simulink model "AStar_Obstacle_Fix_Offset"  (R2019a)
settings: Solver=FixedStepAuto  StartTime=0.0  StopTime=inf  FixedStep=0.1  RelTol=1e-3
undefined symbols (not defined in the file): Angular, Linear
libraries: robotlib x4, simulink x1
settings Model: Creator=user  LastModifiedBy=user
settings OptimizationCC: EnhancedBackFolding=on  PassReuseOutputArgsAs=Individual arguments  MaxStackSize=64  OptimizeBlockOrder=speed  DifferentSizesBufferReuse=on  OptimizationCustomize=off
settings DebuggingCC: ParameterTunabilityLossMsg=error
settings HardwareCC: ProdBitPerPointer=32  ProdBitPerSizeT=32  ProdBitPerPtrDiffT=32  ProdLargestAtomicFloat=None  ProdIntDivRoundTo=Undefined  ProdEndianess=Unspecified  ProdWordSize=32  ProdHWDeviceType=Generic->Unspecified (assume 32-bit Generic)
settings SFSimCC: MATLABDynamicMemAlloc=off
settings RTWCC: SystemTargetFile=ert.tlc  HardwareBoard=Robot Operating System (ROS)  TLCOptions="-aInlineSetEventsForThisBaseRateFcn=TLC_FALSE -aSuppressMultiTaskScheduler=TLC_FALSE  -aRateBasedStepFcn=0"  TemplateMakefile=ert_default_tmf  GenerateReport=on  Toolchain=Catkin  IncludeHyperlinkInReport=on  LaunchReport=on  TargetLang=C++  GenerateTraceInfo=on  GenerateTraceReport=on  GenerateTraceReportSl=on  GenerateTraceReportSf=on  GenerateTraceReportEml=on
settings CodeAppCC: ForceParamTrailComments=on  IgnoreCustomStorageClasses=off  OperatorAnnotations=on  SimulinkDataObjDesc=on  SFDataObjDesc=on  InsertBlockDesc=on

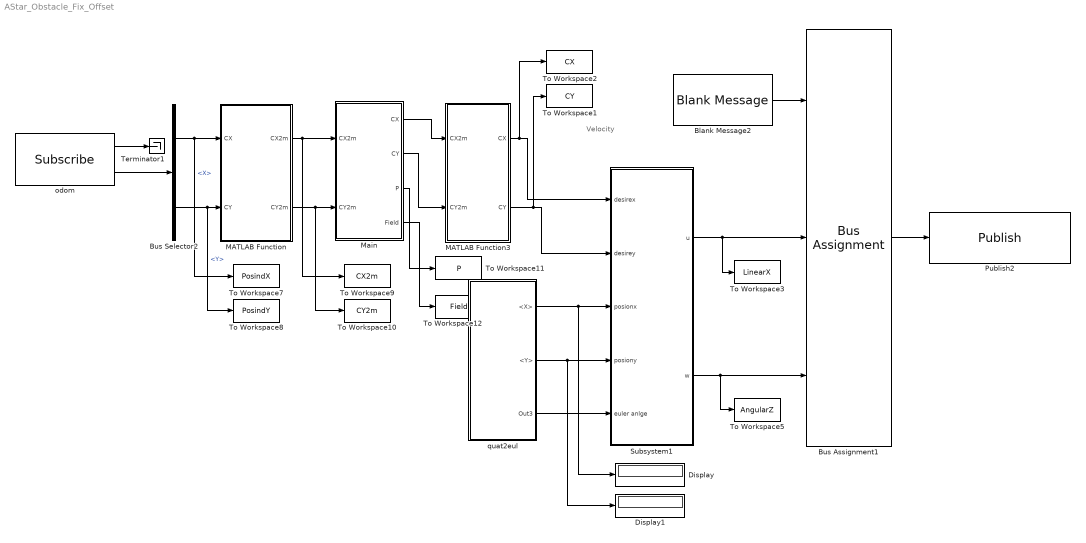
== system AStar_Obstacle_Fix_Offset ==
  note: Velocity
  Blank Message2 : robotlib/Blank Message  messageClass=Message  entityType=geometry_msgs/Twist  messageType=geometry_msgs/Twist  SampleTime=inf
      settings: SourceProductBaseCode=RO
  Bus Assignment1 : BusAssignment  AssignedSignals=Linear.X,Angular.Z
  Bus Selector2 : BusSelector  OutputSignals=Pose.Pose.Position.X,Pose.Pose.Position.Y
  Display : Display
  Display1 : Display
  MATLAB Function : MATLAB Function  TreatAsAtomicUnit=on
  MATLAB Function3 : MATLAB Function  TreatAsAtomicUnit=on
  Main : MATLAB Function  TreatAsAtomicUnit=on
  Publish2 : robotlib/Publish  topicSource=Select from ROS network  topic=/cmd_vel  messageType=geometry_msgs/Twist  messageQueueLength=1
      settings: SourceProductBaseCode=RO
  Subsystem1 : Subsystem
  Terminator1 : Terminator
  To Workspace1 : ToWorkspace  VariableName=CY  SampleTime=-1
      settings: Save2DSignal=2-D array (concatenate along first dimension)
  To Workspace10 : ToWorkspace  VariableName=CY2m  SampleTime=-1
      settings: Save2DSignal=2-D array (concatenate along first dimension)
  To Workspace11 : ToWorkspace  VariableName=P  SampleTime=-1
      settings: Save2DSignal=2-D array (concatenate along first dimension)
  To Workspace12 : ToWorkspace  VariableName=Field  SampleTime=-1
      settings: Save2DSignal=2-D array (concatenate along first dimension)
  To Workspace2 : ToWorkspace  VariableName=CX  SampleTime=-1
      settings: Save2DSignal=2-D array (concatenate along first dimension)
  To Workspace3 : ToWorkspace  VariableName=LinearX  SampleTime=-1
      settings: Save2DSignal=2-D array (concatenate along first dimension)
  To Workspace5 : ToWorkspace  VariableName=AngularZ  SampleTime=-1
      settings: Save2DSignal=2-D array (concatenate along first dimension)
  To Workspace7 : ToWorkspace  VariableName=PosindX  SampleTime=-1
      settings: Save2DSignal=2-D array (concatenate along first dimension)
  To Workspace8 : ToWorkspace  VariableName=PosindY  SampleTime=-1
      settings: Save2DSignal=2-D array (concatenate along first dimension)
  To Workspace9 : ToWorkspace  VariableName=CX2m  SampleTime=-1
      settings: Save2DSignal=2-D array (concatenate along first dimension)
  odom : robotlib/Subscribe  topicSource=Select from ROS network  topic=/odom  messageType=nav_msgs/Odometry  sampleTime=-1  messageQueueLength=1
      settings: SourceProductBaseCode=RO
  quat2eul : Subsystem
  wires:
  MATLAB Function/1(CX2m) -> To Workspace9/1, Main/1(CX2m)
  MATLAB Function/2(CY2m) -> To Workspace10/1, Main/2(CY2m)
  odom/1 -> Terminator1/1
  Main/1(CX) -> MATLAB Function3/1(CX2m)
  Main/2(CY) -> MATLAB Function3/2(CY2m)
  odom/2 -> Bus Selector2/1
  Bus Selector2/1 -> To Workspace7/1, MATLAB Function/1(CX)  "<X>"
  Bus Selector2/2 -> To Workspace8/1, MATLAB Function/2(CY)  "<Y>"
  Subsystem1/2(w) -> To Workspace5/1, Bus Assignment1/3
  quat2eul/2(<Y>) -> Display1/1, Subsystem1/4(posiony)
  MATLAB Function3/1(CX) -> To Workspace2/1, Subsystem1/1(desirex)
  MATLAB Function3/2(CY) -> To Workspace1/1, Subsystem1/2(desirey)
  quat2eul/1(<X>) -> Display/1, Subsystem1/3(posionx)
  Subsystem1/1(u) -> To Workspace3/1, Bus Assignment1/2
  quat2eul/3(Out3) -> Subsystem1/5(euler anlge)
  Bus Assignment1/1 -> Publish2/1
  Blank Message2/1 -> Bus Assignment1/1
  Main/3(P) -> To Workspace11/1
  Main/4(Field) -> To Workspace12/1

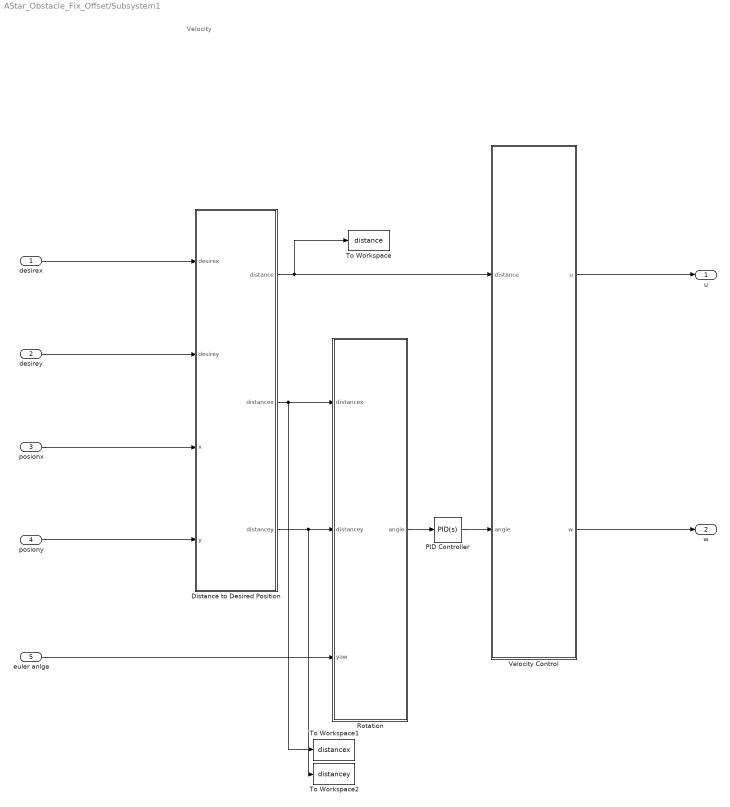
== system AStar_Obstacle_Fix_Offset/Subsystem1 ==
  note: Velocity
  desirex : Inport
  desirey : Inport  Port=2
  posionx : Inport  Port=3
  posiony : Inport  Port=4
  euler anlge : Inport  Port=5
  Distance to Desired Position : MATLAB Function  TreatAsAtomicUnit=on
  PID Controller : simulink/Continuous/PID Controller  Controller=PID  Form=Parallel  TimeDomain=Continuous-time  SampleTime=-1  IntegratorMethod=Forward Euler  FilterMethod=Forward Euler  ControllerParametersSource=internal  P=1.1  I=0  D=0  UseFilter=on  N=100  TunerSelectOption=Transfer Function Based (PID Tuner App)  InitialConditionSource=internal  InitialConditionForIntegrator=0  InitialConditionForFilter=0  DifferentiatorICPrevScaledInput=0  ExternalReset=none  TrackingMode=off  Kt=1  LimitOutput=off  UpperSaturationLimit=inf  LowerSaturationLimit=-inf  LinearizeAsGain=on  AntiWindupMode=none  Kb=1  POutMin=[]  POutMax=[]  IOutMin=[]  IOutMax=[]  DOutMin=[]  DOutMax=[]  NOutMin=[]  NOutMax=[]  SumOutMin=[]  SumOutMax=[]  SaturationOutMin=[]  SaturationOutMax=[]  PParamMin=[]  PParamMax=[]  IParamMin=[]  IParamMax=[]  DParamMin=[]  DParamMax=[]  NParamMin=[]  NParamMax=[]  KbParamMin=[]  KbParamMax=[]  KtParamMin=[]  KtParamMax=[]  KbOutMin=[]  KbOutMax=[]  KtOutMin=[]  KtOutMax=[]  IntegratorOutMin=[]  IntegratorOutMax=[]  FilterOutMin=[]  FilterOutMax=[]  SumI1OutMin=[]  SumI1OutMax=[]  SumI2OutMin=[]  SumI2OutMax=[]  SumI3OutMin=[]  SumI3OutMax=[]  SumI4OutMin=[]  SumI4OutMax=[]  SumDOutMin=[]  SumDOutMax=[]  DifferentiatorOutMin=[]  DifferentiatorOutMax=[]  FilterDiffOutCoefMin=[]  FilterDiffOutCoefMax=[]  ReciprocalOutMin=[]  ReciprocalOutMax=[]  SumDenOutMin=[]  SumDenOutMax=[]  SumNumOutMin=[]  SumNumOutMax=[]  DivideOutMin=[]  DivideOutMax=[]  IntegratorContinuousStateAttributes=''  IntegratorStateMustResolveToSignalObject=off  IntegratorRTWStateStorageClass=Auto  FilterContinuousStateAttributes=''  FilterStateMustResolveToSignalObject=off  FilterRTWStateStorageClass=Auto  ParallelPVariant=InternalParameters  IdealPVariant=Disabled  IVariant=InternalParameters  DVariant=InternalParameters  IntegratorVariant=Continuous  SatVariant=Disabled  AWVariant=Passthrough  PCopyVariant=Disabled  TRVariant=Disabled  FdbkBlocksVariant=Forward  IdealPFdbkVariant=Disabled  SatFdbkVariant=Disabled  DerivativeFilterVariant=ContFilter  NVariant=InternalParameters  NCopyVariant=Disabled  FilterICVariant=InternalICsFilter  IntegratorICVariant=InternalICs  ExternalResetVariant=Disabled  TRSumVariant=Passthrough  SumFdbkVariant=Disabled  SumVariant=Sum_PID
  Rotation : MATLAB Function  TreatAsAtomicUnit=on
  To Workspace : ToWorkspace  VariableName=distance  SampleTime=-1
      settings: Save2DSignal=2-D array (concatenate along first dimension)
  To Workspace1 : ToWorkspace  VariableName=distancex  SampleTime=-1
      settings: Save2DSignal=2-D array (concatenate along first dimension)
  To Workspace2 : ToWorkspace  VariableName=distancey  SampleTime=-1
      settings: Save2DSignal=2-D array (concatenate along first dimension)
  Velocity Control : MATLAB Function  TreatAsAtomicUnit=on
  u : Outport
  w : Outport  Port=2
  wires:
  desirex/1 -> Distance to Desired Position/1(desirex)
  desirey/1 -> Distance to Desired Position/2(desirey)
  Distance to Desired Position/2(distancex) -> To Workspace1/1, Rotation/1(distancex)
  Velocity Control/2(w) -> w/1
  posionx/1 -> Distance to Desired Position/3(x)
  euler anlge/1 -> Rotation/3(yaw)
  posiony/1 -> Distance to Desired Position/4(y)
  Rotation/1(angle) -> PID Controller/1
  PID Controller/1 -> Velocity Control/2(angle)
  Distance to Desired Position/1(distance) -> To Workspace/1, Velocity Control/1(distance)
  Velocity Control/1(u) -> u/1
  Distance to Desired Position/3(distancey) -> To Workspace2/1, Rotation/2(distancey)

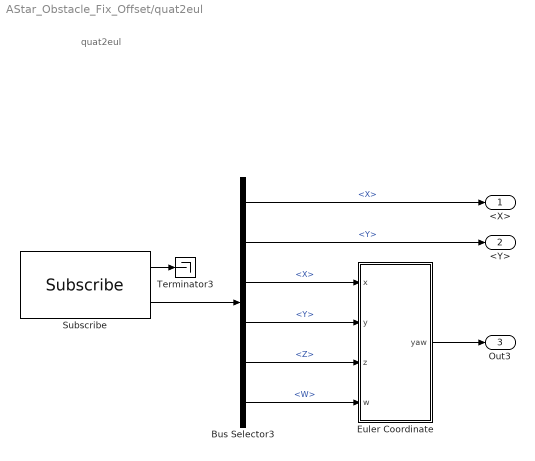
== system AStar_Obstacle_Fix_Offset/quat2eul ==
  note: quat2eul
  Bus Selector3 : BusSelector  OutputSignals=Pose.Pose.Position.X,Pose.Pose.Position.Y,Pose.Pose.Orientation.X,Pose.Pose.Orientation.Y,Pose.Pose.Orientation.Z,Pose.Pose.Orientation.W
  Euler Coordinate : MATLAB Function  TreatAsAtomicUnit=on
  Subscribe : robotlib/Subscribe  topicSource=Select from ROS network  topic=/odom  messageType=nav_msgs/Odometry  sampleTime=-1  messageQueueLength=1
      settings: SourceProductBaseCode=RO
  Terminator3 : Terminator
  <X> : Outport
  <Y> : Outport  Port=2
  Out3 : Outport  Port=3
  wires:
  Euler Coordinate/1(yaw) -> Out3/1
  Bus Selector3/5 -> Euler Coordinate/3(z)  "<Z>"
  Bus Selector3/6 -> Euler Coordinate/4(w)  "<W>"
  Subscribe/1 -> Terminator3/1
  Bus Selector3/3 -> Euler Coordinate/1(x)  "<X>"
  Subscribe/2 -> Bus Selector3/1
  Bus Selector3/4 -> Euler Coordinate/2(y)  "<Y>"
  Bus Selector3/2 -> <Y>/1  "<Y>"
  Bus Selector3/1 -> <X>/1  "<X>"

== matlab function AStar_Obstacle_Fix_Offset/quat2eul/Euler Coordinate ==
  data: x input; yaw output; y input; z input; w input
function yaw = quat2eul(x,y,z,w)

eul = quat2eul([w,x,y,z]);
yaw = eul(1);

end

== matlab function AStar_Obstacle_Fix_Offset/Main ==
  data: CX2m input; CY2m input; CX output; CY output; P output; Field output
function [CX,CY,P,Field] = astar(CX2m,CY2m)

N = 35;
Look = 0.04;
Offset = 50;

Start = [CY2m,CX2m]; % 반대로 줘야 함
Goal = [31,31]; % 반대로 줘야 함

Field = ones(N,N);
Step = round(N/4);
ObstacleRange = 3;

% 테두리
Field(1:ObstacleRange,:) = Inf;
Field(N-ObstacleRange:N,:) = Inf;
Field(:,1:ObstacleRange) = Inf;
Field(:,N-ObstacleRange:N) = Inf;
% 가로 장애물
Field(Step-ObstacleRange:Step+ObstacleRange,N-Step-ObstacleRange:N) = Inf;
Field(Step*2-ObstacleRange:Step*2+ObstacleRange,1:Step+ObstacleRange) = Inf;
Field(Step*2-ObstacleRange:Step*2+ObstacleRange,N-Step-ObstacleRange:N) = Inf;
Field(Step*3-ObstacleRange:Step*3+ObstacleRange,1:Step+ObstacleRange) = Inf;
Field(Step*3-ObstacleRange:Step*3+ObstacleRange,N-Step-ObstacleRange:N) = Inf;
% 세로 장애물
Field(1:Step+ObstacleRange,Step-ObstacleRange:Step+ObstacleRange) = Inf;
Field(Step-ObstacleRange:Step*2+ObstacleRange,Step*2-ObstacleRange:Step*2+ObstacleRange) = Inf;
Field(N-Step-ObstacleRange:N,Step*2-ObstacleRange:Step*2+ObstacleRange) = Inf;

FScore = inf(N,N);
FScore(Start(1),Start(2)) = 0;
GScore = inf(N,N);
GScore(Start(1),Start(2)) = 0;
HScore = inf(N,N);
Fieldpointers = inf(N,N); % 1 2 3 4중 하나가 기록되어 부모노드의 방향을 기록
Fieldpointers(Start(1),Start(2)) = 0; % 0은 출발점을 의미
Fieldpointers(Goal(1),Goal(2)) = 0; % 도착점이 0이었다가 0이 아니게 되면 반복 종료.
Movementnumber = [1 2 3 4]; % 1:Up 2:Right 3:Bottom 4:Right

figure(1);
[i,j] = find(Field==1);
plot(j,i,'*');
set(gca,'Xlim',[0,N],'Ylim',[0,N]);
xlabel('X');
ylabel('Y');

% G(x)
G_top = [inf 1 inf];
G_mid = [1 0 1];
G_bottom = [inf 1 inf];

% Define Heuristic

for i=1:N
    for j=1:N
        HScore(i,j) = (abs(i-Start(1)) + abs(j-Start(2)))*1;
    end
end

% AStar
while Fieldpointers(Goal(1),Goal(2)) == 0
    if Start(1) == Goal(1) && Start(2) == Goal(2)
        break;
    end
    [minFScore,~] = min(min(FScore));
    [i_x,j_y] = find(FScore==minFScore);

    i = i_x(1);
    j = j_y(1);
    
    if Field(i,j+1) ~= inf
        if min(GScore(i,j+1),GScore(i,j)+G_top(1,2)) == GScore(i,j+1)
            Fieldpointers(i,j+1) = Fieldpointers(i,j+1); % Stay
        else
            Fieldpointers(i,j+1) = Movementnumber(1); % Up
        end
        GScore(i,j+1) = min(GScore(i,j+1),GScore(i,j)+G_top(1,2)); % Up
    end
    
    if Field(i+1,j) ~= inf
        if min(GScore(i+1,j),GScore(i,j)+G_mid(1,3)) == GScore(i+1,j)
            Fieldpointers(i+1,j) = Fieldpointers(i+1,j);
        else
            Fieldpointers(i+1,j) = Movementnumber(2); % Right
        end
        GScore(i+1,j) = min(GScore(i+1,j),GScore(i,j)+G_mid(1,3)); % Right
    end
    
    if Field(i,j-1) ~= inf
        if min(GScore(i,j-1),GScore(i,j)+G_bottom(1,2)) == GScore(i,j-1)
            Fieldpointers(i,j-1) = Fieldpointers(i,j-1);
        else
            Fieldpointers(i,j-1) = Movementnumber(3); % Down
        end
        GScore(i,j-1) = min(GScore(i,j-1),GScore(i,j)+G_bottom(1,2)); % Down
    end
    
    if Field(i-1,j) ~= inf
        if min(GScore(i-1,j),GScore(i,j)+G_mid(1,1)) == GScore(i-1,j)
            Fieldpointers(i-1,j) = Fieldpointers(i-1,j);
        else
            Fieldpointers(i-1,j) = Movementnumber(4); % Left
        end
        GScore(i-1,j) = min(GScore(i-1,j),GScore(i,j)+G_mid(1,1)); % Left
    end
   
    FScore = GScore + HScore;
    Field(i,j) = inf;
    FScore(Field==inf) = inf;
end

%
Search = Goal;
P = zeros(100,2);
for i=1:100
    P(i,:) = Search;
    if Fieldpointers(Search(1),Search(2)) == 1
        Search = [Search(1),Search(2)-1];
    elseif Fieldpointers(Search(1),Search(2)) == 2
        Search = [Search(1)-1,Search(2)];
    elseif Fieldpointers(Search(1),Search(2)) == 3
        Search = [Search(1),Search(2)+1];
    elseif Fieldpointers(Search(1),Search(2)) == 4
        Search = [Search(1)+1,Search(2)];
    else
        break;
    end
end

figure(2);
plot(P(:,2),P(:,1),'*');
set(gca,'Xlim',[0,N],'Ylim',[0,N]);
xlabel('X');
ylabel('Y');

if P(i,2) == Goal(2) && P(i,1) == Goal(1)
    CX = P(i,2);
    CY = P(i,1);
else
    CX = P(i-1,2);
    CY = P(i-1,1);
end

== matlab function AStar_Obstacle_Fix_Offset/Subsystem1/Velocity Control ==
  data: distance input; u output; angle input; w output
function [u,w] = velocity(distance,angle)

if (angle <= 0.05) && (angle >= -0.05)
    u = 0.05;
    if (distance <= 0.015)
        u = 0;
    end
else
    u = 0;
end

w = angle;

== matlab function AStar_Obstacle_Fix_Offset/Subsystem1/Rotation ==
  data: distancex input; angle output; distancey input; yaw input
function angle = angle(distancex,distancey,yaw)

desireangle = atan2(distancey,distancex);
u = desireangle - yaw;
angle =  atan2(sin(u),cos(u));

== matlab function AStar_Obstacle_Fix_Offset/Subsystem1/Distance to Desired Position ==
  data: distance output; desirex input; distancex output; desirey input; x input; y input; distancey output
function [distance,distancex,distancey] = distance(desirex,desirey,x,y)

distancex = desirex - x;
distancey = desirey - y;
distance = sqrt(distancex^2 + distancey^2);

== matlab function AStar_Obstacle_Fix_Offset/MATLAB Function ==
  data: CX input; CX2m output; CY input; CY2m output
function [CX2m,CY2m] = carte2mat(CX,CY)
% 실제 위치를 행렬 위치로 바꾼다.

persistent Memory_X Memory_Y;

if isempty(Memory_X)
    Memory_X = 0;
    Memory_Y = 0;
end

Look = 0.04; % 팬스의 길이 단위
Height = 35; % 미로 전체에서 x축에 필요한 팬스 갯수
Width = 35; % y축에 필요한 팬스 갯수
Start = [4,4];

n1 = 0;
n2 = 0;
ir = 0;
for i=1:Height
    if (CX >= n1-0.02) && (CX <= n1+0.02)
        CX2m = i+(Start(1)-1);
        Memory_X = i+(Start(1)-1);
        break;
    end
    if (CX >= n2-0.02) && (CX <= n2+0.02)
        CX2m = ir+(Start(1));
        Memory_X = ir+(Start(1));
        break;
    end
    n1 = n1 + Look;
    n2 = n2 - Look;
    ir = ir - 1;
    CX2m = Memory_X;
end

n1 = 0;
n2 = 0;
jr = 0;
for j=1:Width
    if (CY >= n1-0.02) && (CY <= n1+0.02)
        CY2m = j+(Start(2)-1);
        Memory_Y = j+(Start(2)-1);
        break;
    end
    if (CY >= n2-0.02) && (CY <= n2+0.02)
        CY2m = jr+(Start(2));
        Memory_Y = jr+(Start(2));
        break;
    end
    n1 = n1 + Look;
    n2 = n2 - Look;
    jr = jr - 1;
    CY2m = Memory_Y;
end

== matlab function AStar_Obstacle_Fix_Offset/MATLAB Function3 ==
  data: CX2m input size=1; CX output; CY2m input size=1; CY output
function [CX,CY] = mat2carte(CX2m,CY2m)
% 행렬 위치를 실제 위치로 바꾼다.

Look = 0.04; % 1개 노드의 단위
Start = [4,4];

CX = (CX2m-(Start(1))) * Look;
CY = (CY2m-(Start(2))) * Look;
